simulink model "PID_Controller_with_delay"  (R2014b)
settings: Solver=ode45  StartTime=0.0  StopTime=20  RelTol=1e-3
undefined symbols (not defined in the file or in its folder): fdesignblkfcn, gcbh, sigbuilder_block
libraries: simulink x3
settings Model: Creator=Asus  LastModifiedBy=Asus

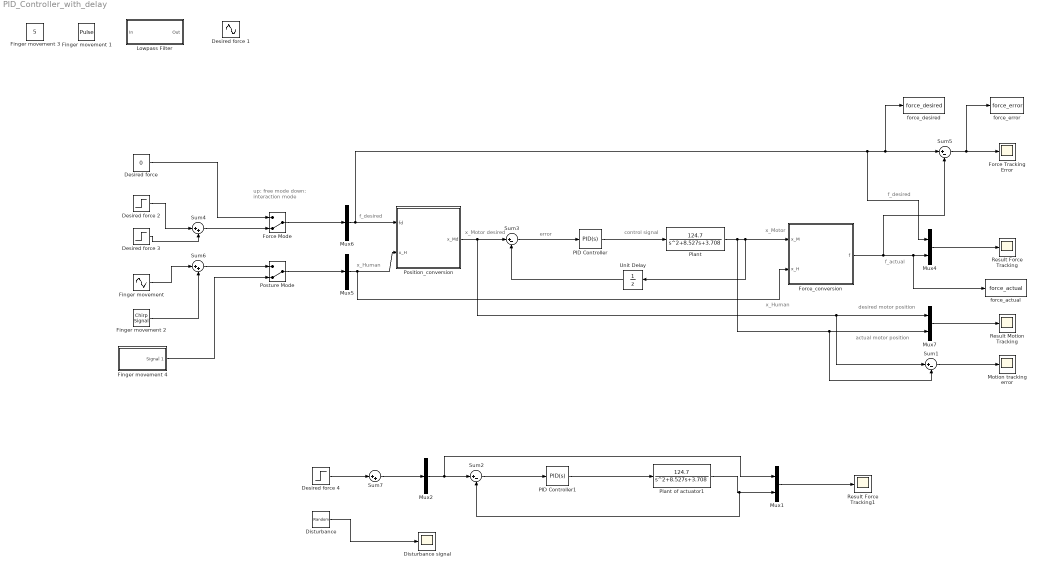
== system PID_Controller_with_delay ==
  note: up: free mode
      | down: interaction mode
  note: control signal
  note: error
  note: x_Motor
  note: x_Motor desired
  note: x_Human
  note: actual motor position
  note: desired motor position
  note: f_desired
  note: f_actual
  note: x_Human
  note: f_desired
  Desired force : Constant  Value=0
  Desired force 1 : Sin  Samples=20  SampleTime=0
  Desired force 2 : Step  Time=3  After=5  SampleTime=0
  Desired force 3 : Step  Time=6  After=-5  SampleTime=0
  Desired force 4 : Step  SampleTime=0
  Disturbance : RandomNumber  Variance=0.1  Seed=0.1  SampleTime=0.05
  Disturbance signal : Scope
      settings: TickLabels=on  ShowLegends=on  SaveName=Result_Force_Tracking2
  Finger movement 1 : DiscretePulseGenerator  PulseType=Time based  Period=5  PulseWidth=50
  Finger movement : Sin  Bias=8  Frequency=2  Samples=20  SampleTime=0
  Finger movement 2 : simulink/Sources/Chirp Signal  f1=0  T=20  f2=1
  Finger movement 3 : Constant  Value=5
  Finger movement 4 : Subsystem  Tag=STV Subsys  LoadFcn=sigbuilder_block('load');  StartFcn=sigbuilder_block('start');  StopFcn=sigbuilder_block('stop');  ClipboardFcn=sigbuilder_block('clipboard');  mask(Sigbuilder block){}
      mask help: Simulink:masks:SigbuilderBlock_MD
      mask init:
      | if ~strcmp(get_param(bdroot(gcbh),'SimulationStatus'),'stopped') tuvar = sigbuilder_block('maskInit'); end
      settings: CopyFcn=sigbuilder_block('copy');  DeleteFcn=sigbuilder_block('delete');  ModelCloseFcn=sigbuilder_block('modelClose');  PreSaveFcn=sigbuilder_block('preSave');  PauseFcn=sigbuilder_block('pause');  ContinueFcn=sigbuilder_block('continue');  NameChangeFcn=sigbuilder_block('namechange');  OpenFcn=sigbuilder_block('open',[437.6 199.2 550.4 400 ]);  CloseFcn=sigbuilder_block('close');
      mask Display: plot(0, 0, 100, 100,[2, 2, 32, 32, 2], [68, 8, 8, 68, 68],[32, 2], [38, 38], [32, 19, 2],[53, 60, 44], [32, 17, 17, 2],[16, 16, 31, 31]);txt = getActiveGroup(gcbh);text(2, 100, txt,'verticalAlignment', 'top');
  Force Mode : ManualSwitch  CurrentSetting=0
  Force Tracking Error : Scope
      settings: ShowLegends=on  TimeRange=20  YMin=-5.005624140355663  SaveName=ScopeData5
  Force_conversion : MATLAB Function  TreatAsAtomicUnit=on
  Lowpass Filter : Subsystem  DialogController=fdesignblkfcn  InitFcn=fdesignblkfcn(gcbh, {'InitFcn'});  mask(Lowpass Filter){}
      mask help: Design a lowpass filter
      settings: CopyFcn=fdesignblkfcn(gcbh, {'CopyFcn'});
      mask Help: helpview(mapfilelocation('dsp'), 'dsplowpassfilter');
      mask Display: disp('Lowpass')
  Motion tracking error : Scope
      settings: ShowLegends=on
  Mux1 : Mux  Inputs=2
  Mux2 : Mux  Inputs=1
  Mux4 : Mux  Inputs=2
  Mux5 : Mux  Inputs=1
  Mux6 : Mux  Inputs=1
  Mux7 : Mux  Inputs=2
  PID Controller : simulink/Continuous/PID Controller  Controller=PID  TimeDomain=Continuous-time  SampleTime=-1  IntegratorMethod=Forward Euler  FilterMethod=Forward Euler  Form=Parallel  P=0.692993618695865  I=0.279691466170031  D=0.0929069207502412  N=22.22989187167  InitialConditionSource=internal  InitialConditionForIntegrator=0  InitialConditionForFilter=0  ExternalReset=none  LimitOutput=off  UpperSaturationLimit=inf  LowerSaturationLimit=-inf  LinearizeAsGain=on  AntiWindupMode=none  Kb=1  TrackingMode=off  Kt=1  PParamMin=[]  PParamMax=[]  IParamMin=[]  IParamMax=[]  DParamMin=[]  DParamMax=[]  NParamMin=[]  NParamMax=[]  KbParamMin=[]  KbParamMax=[]  KtParamMin=[]  KtParamMax=[]  POutMin=[]  POutMax=[]  IOutMin=[]  IOutMax=[]  DOutMin=[]  DOutMax=[]  NOutMin=[]  NOutMax=[]  KbOutMin=[]  KbOutMax=[]  KtOutMin=[]  KtOutMax=[]  IntegratorOutMin=[]  IntegratorOutMax=[]  FilterOutMin=[]  FilterOutMax=[]  SumOutMin=[]  SumOutMax=[]  SumI1OutMin=[]  SumI1OutMax=[]  SumI2OutMin=[]  SumI2OutMax=[]  SumI3OutMin=[]  SumI3OutMax=[]  SumDOutMin=[]  SumDOutMax=[]  SaturationOutMin=[]  SaturationOutMax=[]  IntegratorContinuousStateAttributes=''  IntegratorStateMustResolveToSignalObject=off  IntegratorRTWStateStorageClass=Auto  FilterContinuousStateAttributes=''  FilterStateMustResolveToSignalObject=off  FilterRTWStateStorageClass=Auto  DifferentiatorICPrevScaledInput=0  DifferentiatorOutMin=[]  DifferentiatorOutMax=[]  UseFilter=on
  PID Controller1 : simulink/Continuous/PID Controller  Controller=PID  TimeDomain=Continuous-time  SampleTime=-1  IntegratorMethod=Forward Euler  FilterMethod=Forward Euler  Form=Parallel  P=0.592993618695865  I=0.279691466170031  D=0.0429069207502412  N=22.22989187167  InitialConditionSource=internal  InitialConditionForIntegrator=0  InitialConditionForFilter=0  ExternalReset=none  LimitOutput=off  UpperSaturationLimit=inf  LowerSaturationLimit=-inf  LinearizeAsGain=on  AntiWindupMode=none  Kb=1  TrackingMode=off  Kt=1  PParamMin=[]  PParamMax=[]  IParamMin=[]  IParamMax=[]  DParamMin=[]  DParamMax=[]  NParamMin=[]  NParamMax=[]  KbParamMin=[]  KbParamMax=[]  KtParamMin=[]  KtParamMax=[]  POutMin=[]  POutMax=[]  IOutMin=[]  IOutMax=[]  DOutMin=[]  DOutMax=[]  NOutMin=[]  NOutMax=[]  KbOutMin=[]  KbOutMax=[]  KtOutMin=[]  KtOutMax=[]  IntegratorOutMin=[]  IntegratorOutMax=[]  FilterOutMin=[]  FilterOutMax=[]  SumOutMin=[]  SumOutMax=[]  SumI1OutMin=[]  SumI1OutMax=[]  SumI2OutMin=[]  SumI2OutMax=[]  SumI3OutMin=[]  SumI3OutMax=[]  SumDOutMin=[]  SumDOutMax=[]  SaturationOutMin=[]  SaturationOutMax=[]  IntegratorContinuousStateAttributes=''  IntegratorStateMustResolveToSignalObject=off  IntegratorRTWStateStorageClass=Auto  FilterContinuousStateAttributes=''  FilterStateMustResolveToSignalObject=off  FilterRTWStateStorageClass=Auto  DifferentiatorICPrevScaledInput=0  DifferentiatorOutMin=[]  DifferentiatorOutMax=[]  UseFilter=on
  Plant : TransferFcn  Numerator=[124.7]  Denominator=[1 8.527 3.708]
  Plant of actuator1 : TransferFcn  Numerator=[124.7]  Denominator=[1 8.527 3.708]
  Position_conversion : MATLAB Function  TreatAsAtomicUnit=on
  Posture Mode : ManualSwitch  CurrentSetting=0
  Result Force Tracking : Scope
      settings: TickLabels=on  ShowLegends=on  SaveName=Result_Force_Tracking
  Result Force Tracking1 : Scope
      settings: TickLabels=on  ShowLegends=on  SaveName=Result_Force_Tracking1
  Result Motion Tracking : Scope
      settings: ShowLegends=on  SaveName=Result_Motion_Tracking
  Sum{1..3,5} (4 alike) : Sum  Inputs=|+-
  Sum4 : Sum  Inputs=|++
  Sum6 : Sum  Inputs=|++
  Sum7 : Sum  Inputs=|++
  Unit Delay : UnitDelay  SampleTime=-1
  "force_actual " : ToWorkspace  VariableName=force_actual  SampleTime=-1
      settings: Save2DSignal=2-D array (concatenate along first dimension)
  force_desired : ToWorkspace  VariableName=force_desired  SampleTime=-1
      settings: Save2DSignal=2-D array (concatenate along first dimension)
  force_error : ToWorkspace  VariableName=force_error  SampleTime=-1
      settings: Save2DSignal=2-D array (concatenate along first dimension)
  wires:
  Position_conversion/1(x_Md) -> Sum1/1, Mux7/1, Sum3/1
  Plant/1 -> Sum1/2, Mux7/2, Unit Delay/1, Force_conversion/1(x_M)
  Force_conversion/1(f) -> Sum5/2, "force_actual "/1, Mux4/2
  Mux5/1 -> Force_conversion/2(x_H), Position_conversion/2(x_H)
  Mux6/1 -> Mux4/1, force_desired/1, Sum5/1, Position_conversion/1(fd)
  Mux7/1 -> Result Motion Tracking/1
  Sum5/1 -> force_error/1, Force Tracking Error/1
  Mux4/1 -> Result Force Tracking/1
  Sum1/1 -> Motion tracking error/1
  Desired force 3/1 -> Sum4/2
  Desired force 2/1 -> Sum4/1
  Sum3/1 -> PID Controller/1
  PID Controller/1 -> Plant/1
  Sum2/1 -> PID Controller1/1
  PID Controller1/1 -> Plant of actuator1/1
  Mux1/1 -> Result Force Tracking1/1
  Plant of actuator1/1 -> Sum2/2, Mux1/2
  Finger movement 4/1(Signal 1) -> Posture Mode/2
  Force Mode/1 -> Mux6/1
  Posture Mode/1 -> Mux5/1
  Desired force/1 -> Force Mode/1
  Finger movement/1 -> Sum6/1
  Sum6/1 -> Posture Mode/1
  Finger movement 2/1 -> Sum6/2
  Disturbance/1 -> Disturbance signal/1
  Desired force 4/1 -> Sum7/1
  Sum7/1 -> Mux2/1
  Mux2/1 -> Mux1/1, Sum2/1
  Sum4/1 -> Force Mode/2
  Unit Delay/1 -> Sum3/2

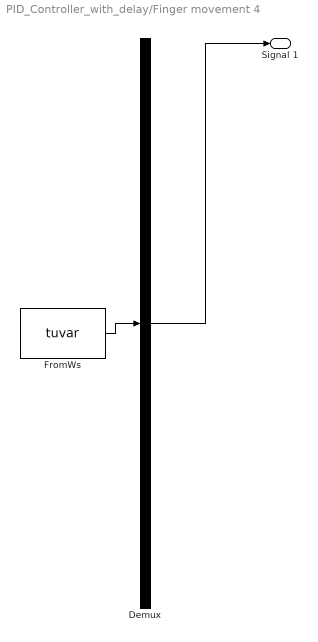
== system PID_Controller_with_delay/Finger movement 4 ==
  Demux : Demux  Tag=STV Demux  Outputs=1
  FromWs : FromWorkspace  Tag=STV FromWs  VariableName=tuvar  SampleTime=0
      SigBuilderData=|
      | common.afterFinalStr = 'Extrapolate'
      | common.sampleTime = 0
      | dataSet.timeRange = [0 10]
      | dataSet.name = 'Group 1'
      | sbobj.Groups.Name = 'Group 1'
      | sbobj.Groups.Signals.Name = 'Signal 1'
      | sbobj.Groups.Signals.XData = [0 3 6 10]
      | sbobj.Groups.Signals.YData = [8 13 13 8]
  Signal 1 : Outport  Tag=STV Outport
  wires:
  Demux/1 -> Signal 1/1
  FromWs/1 -> Demux/1

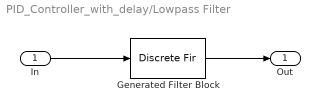
== system PID_Controller_with_delay/Lowpass Filter ==
  In : Inport
  Generated Filter Block : DiscreteFir  Tag=BlockMethodSubSystem  Coefficients=[-0.0024228738523269194 -0.0020832449820793156 0.0067703446401186319 0.01673194542348903 0.011117076081077624 -0.006231145414144477 -0.0084016171860268381 0.0092567976151380574 0.012982883808855736 -0.010121234703278957 -0.018273518733782464 0.011431962071777983 0.02617588858040763 -0.012489027835322955 -0.037996623145463627 0.013388945199366925 0.05815546581472987 -0.014048043515808928 -0.10272466857882168 0.014462275771238398 0.31716649721769485 0.48538764678732504 0.31716649721769485 0.014462275771238398 -0.10272466857882168 -0.014048043515808928 0.05815546581472987 0.013388945199366925 -0.037996623145463627 -0.012489027835322955 0.02617588858040763 0.011431962071777983 -0.018273518733782464 -0.010121234703278957 0.012982883808855736 0.0092567976151380574 -0.0084016171860268381 -0.006231145414144477 0.011117076081077624 0.01673194542348903 0.0067703446401186319 -0.0020832449820793156 -0.0024228738523269194]  InputProcessing=Columns as channels (frame based)
  Out : Outport
  wires:
  In/1 -> Generated Filter Block/1
  Generated Filter Block/1 -> Out/1

== matlab function PID_Controller_with_delay/Force_conversion ==
  data: x_M input; f output; x_H input
function f = force_conver(x_M,x_H)
%#codegen
    k = 0.434;
    L0 = 8;
    f = k*(x_H - x_M - L0);
end

== matlab function PID_Controller_with_delay/Position_conversion ==
  data: fd input; x_Md output; x_H input
function x_Md = pos_conver(fd,x_H)
%#codegen
    k = 0.434; %N/mm
    L0 = 8;    %mm
    x_Md = x_H - (fd/k) - L0;
end
